simulink model "mode_controller"  (R2017a)
settings: Solver=VariableStepAuto  StartTime=0.0  StopTime=inf  RelTol=1e-3
settings Model: Creator=mini  LastModifiedBy=mini

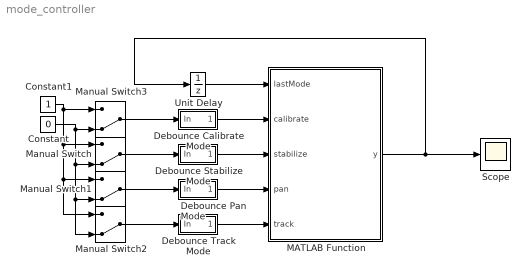
== system mode_controller ==
  Constant : Constant  Value=0
  Constant1 : Constant
  Debounce Calibrate Mode : Subsystem  TreatAsAtomicUnit=on  mask(Debounce){debounce_count=20}
      mask prompts: debounce_count "Debounce count"
      mask help: Number of consecutive samples before changing states.
  Debounce Pan Mode : Subsystem  TreatAsAtomicUnit=on  mask(Debounce){debounce_count=20}
      mask prompts: debounce_count "Debounce count"
      mask help: Number of consecutive samples before changing states.
  Debounce Stabilize Mode : Subsystem  TreatAsAtomicUnit=on  mask(Debounce){debounce_count=20}
      mask prompts: debounce_count "Debounce count"
      mask help: Number of consecutive samples before changing states.
  Debounce Track Mode : Subsystem  TreatAsAtomicUnit=on  mask(Debounce){debounce_count=20}
      mask prompts: debounce_count "Debounce count"
      mask help: Number of consecutive samples before changing states.
  MATLAB Function : MATLAB Function  TreatAsAtomicUnit=on
  Manual Switch{,1..3} (4 alike) : ManualSwitch  CurrentSetting=0
  Scope : Scope
  Unit Delay : UnitDelay  SampleTime=-1
  wires:
  Manual Switch/1 -> Debounce Stabilize Mode/1(In)
  Manual Switch2/1 -> Debounce Track Mode/1(In)
  Manual Switch3/1 -> Debounce Calibrate Mode/1(In)
  Manual Switch1/1 -> Debounce Pan Mode/1(In)
  Constant/1 -> Manual Switch3/2, Manual Switch2/2, Manual Switch1/2, Manual Switch/2
  Constant1/1 -> Manual Switch3/1, Manual Switch2/1, Manual Switch1/1, Manual Switch/1
  MATLAB Function/1(y) -> Unit Delay/1, Scope/1
  Unit Delay/1 -> MATLAB Function/1(lastMode)
  Debounce Track Mode/1(Out) -> MATLAB Function/5(track)
  Debounce Pan Mode/1(Out) -> MATLAB Function/4(pan)
  Debounce Stabilize Mode/1(Out) -> MATLAB Function/3(stabilize)
  Debounce Calibrate Mode/1(Out) -> MATLAB Function/2(calibrate)

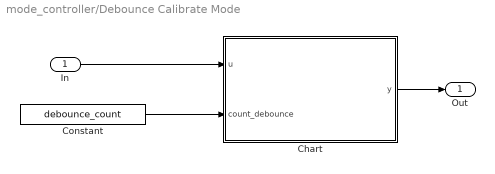
== system mode_controller/Debounce Calibrate Mode ==
  In : Inport
  Chart : Stateflow chart  TreatAsAtomicUnit=on
  Constant : Constant  Value=debounce_count  OutDataTypeStr=uint8  SampleTime=-1
  Out : Outport
  wires:
  In/1 -> Chart/1(u)
  Chart/1(y) -> Out/1
  Constant/1 -> Chart/2(count_debounce)

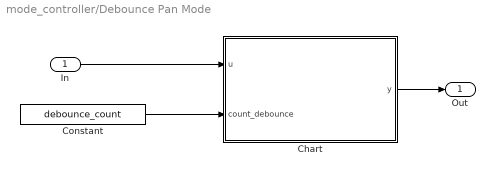
== system mode_controller/Debounce Pan Mode ==
  In : Inport
  Chart : Stateflow chart  TreatAsAtomicUnit=on
  Constant : Constant  Value=debounce_count  OutDataTypeStr=uint8  SampleTime=-1
  Out : Outport
  wires:
  In/1 -> Chart/1(u)
  Chart/1(y) -> Out/1
  Constant/1 -> Chart/2(count_debounce)

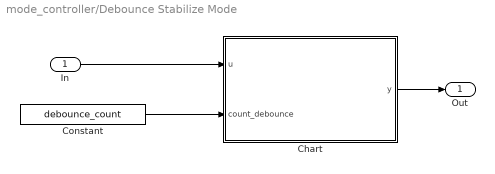
== system mode_controller/Debounce Stabilize Mode ==
  In : Inport
  Chart : Stateflow chart  TreatAsAtomicUnit=on
  Constant : Constant  Value=debounce_count  OutDataTypeStr=uint8  SampleTime=-1
  Out : Outport
  wires:
  In/1 -> Chart/1(u)
  Chart/1(y) -> Out/1
  Constant/1 -> Chart/2(count_debounce)

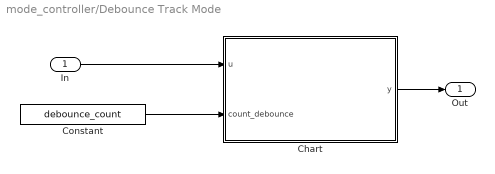
== system mode_controller/Debounce Track Mode ==
  In : Inport
  Chart : Stateflow chart  TreatAsAtomicUnit=on
  Constant : Constant  Value=debounce_count  OutDataTypeStr=uint8  SampleTime=-1
  Out : Outport
  wires:
  In/1 -> Chart/1(u)
  Chart/1(y) -> Out/1
  Constant/1 -> Chart/2(count_debounce)

== stateflow chart mode_controller/Debounce Calibrate Mode/Chart ==
  settings: executeAtInitialization=1
  (default) -> (junction 2)
  (junction 2) -> (junction 3) [order 1] : [u == u_n1]
  (junction 2) -> (junction 13) [order 2] : {count = 0;}
  (junction 3) -> (junction 5)
  (junction 5) -> (junction 7) [order 1] : [count >= count_debounce]
  (junction 7) -> (junction 9) : {y = u;}
  (junction 5) -> (junction 11) [order 2] : {count = count + 1;}
  (junction 11) -> (junction 13)
  (junction 9) -> (junction 11)
  (junction 13) -> (junction 17) : {u_n1 = u;}
  data: u input; u_n1 local type(u); y output type(u); count local uint8; count_debounce input

== matlab function mode_controller/MATLAB Function ==
  data: lastMode input; y output; calibrate input; stabilize input; pan input; track input
function y = fcn(lastMode, calibrate, stabilize, pan, track)
    % default action on startup 
    % TODO add OFF mode?
    if ( calibrate || lastMode == 0 )
        mode = 1;
    elseif ( stabilize )
        mode = 2;
    elseif ( pan )
        mode = 3;
    elseif ( track )
        mode = 4;
    else
        mode = lastMode;
    end
y = mode;

== stateflow chart mode_controller/Debounce Pan Mode/Chart ==
  settings: executeAtInitialization=1
  (default) -> (junction 2)
  (junction 2) -> (junction 3) [order 1] : [u == u_n1]
  (junction 2) -> (junction 13) [order 2] : {count = 0;}
  (junction 3) -> (junction 5)
  (junction 5) -> (junction 7) [order 1] : [count >= count_debounce]
  (junction 7) -> (junction 9) : {y = u;}
  (junction 5) -> (junction 11) [order 2] : {count = count + 1;}
  (junction 11) -> (junction 13)
  (junction 9) -> (junction 11)
  (junction 13) -> (junction 17) : {u_n1 = u;}
  data: u input; u_n1 local type(u); y output type(u); count local uint8; count_debounce input

== stateflow chart mode_controller/Debounce Stabilize Mode/Chart ==
  settings: executeAtInitialization=1
  (default) -> (junction 2)
  (junction 2) -> (junction 3) [order 1] : [u == u_n1]
  (junction 2) -> (junction 13) [order 2] : {count = 0;}
  (junction 3) -> (junction 5)
  (junction 5) -> (junction 7) [order 1] : [count >= count_debounce]
  (junction 7) -> (junction 9) : {y = u;}
  (junction 5) -> (junction 11) [order 2] : {count = count + 1;}
  (junction 11) -> (junction 13)
  (junction 9) -> (junction 11)
  (junction 13) -> (junction 17) : {u_n1 = u;}
  data: u input; u_n1 local type(u); y output type(u); count local uint8; count_debounce input

== stateflow chart mode_controller/Debounce Track Mode/Chart ==
  settings: executeAtInitialization=1
  (default) -> (junction 2)
  (junction 2) -> (junction 3) [order 1] : [u == u_n1]
  (junction 2) -> (junction 13) [order 2] : {count = 0;}
  (junction 3) -> (junction 5)
  (junction 5) -> (junction 7) [order 1] : [count >= count_debounce]
  (junction 7) -> (junction 9) : {y = u;}
  (junction 5) -> (junction 11) [order 2] : {count = count + 1;}
  (junction 11) -> (junction 13)
  (junction 9) -> (junction 11)
  (junction 13) -> (junction 17) : {u_n1 = u;}
  data: u input; u_n1 local type(u); y output type(u); count local uint8; count_debounce input
